simulink model "my_simslx"  (R2020b)
settings: Solver=VariableStepAuto  StartTime=0.0  StopTime=10.0  RelTol=1e-3
settings Model: Creator=Sugusokothx  LastModifiedBy=Sugusokothx
settings SFSimCC: SimCustomHeaderCode="#include \"Main.h\""  SimUserSources=Main.c const.c myAdd.c mySub.c  SimUserIncludeDirs=./src

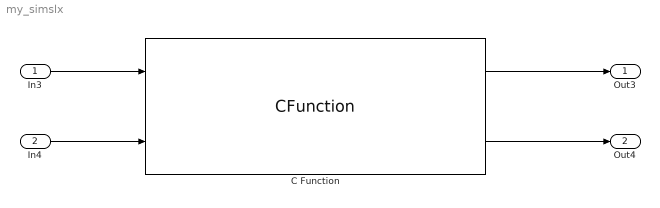
== system my_simslx ==
  In3 : Inport
  In4 : Inport  Port=2
  C Function : CFunction  OutputCode=Main2(u1, u2, &y1, &y2);
  Out3 : Outport
  Out4 : Outport  Port=2
  wires:
  C Function/1 -> Out3/1
  In3/1 -> C Function/1
  C Function/2 -> Out4/1
  In4/1 -> C Function/2
